simulink subsystem "BatteryHVElectrical_refsub"  (R2022a)
settings: Solver=VariableStepAuto  StartTime=0.0  StopTime=10.0  RelTol=1e-3
undefined symbols (not defined in the file): batteryHighVoltage, Minus, Plus
libraries: fl_lib x7, nesl_utility x6, ee_lib x1
settings Model: Creator=isaacito  LastModifiedBy=isaacito
settings SolverCC: AlgebraicLoopSolver=TrustRegion
settings DebuggingCC: UnconnectedInputMsg=warning  UnconnectedOutputMsg=warning  UnconnectedLineMsg=warning  SFMachineParentedDataDiag=warning
settings RTWCC: DLArmComputeVersion=19.05

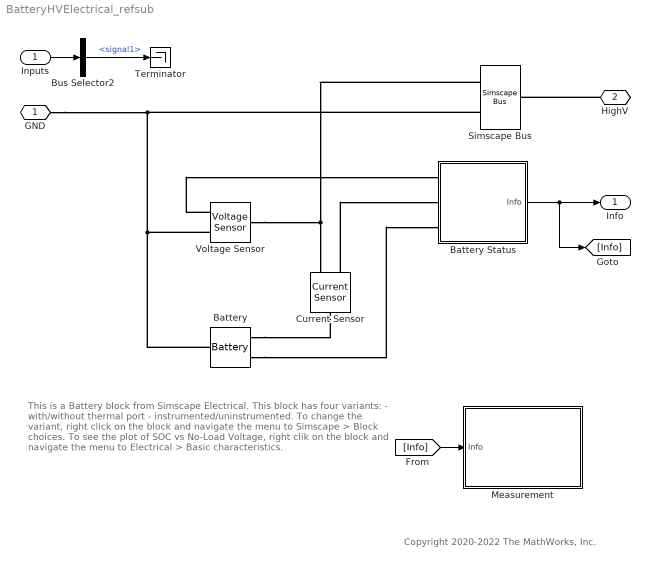
== system BatteryHVElectrical_refsub ==
  note: This is a Battery block from Simscape Electrical.
      | This block has four variants:
      | - with/without thermal port
      | - instrumented/uninstrumented.
      | To change the variant, right click on the block and
      | navigate the menu to Simscape > Block choices.
      |
      | To see the plot of SOC vs No-Load Voltage,
      | right clik on the block and navigate the menu
      | to Electrical > Basic characteristics.
  note: Copyright 2020-2022 The MathWorks, Inc.
  Inputs : Inport
  Battery : ee_lib/Sources/Battery  Vnom=batteryHighVoltage.packVoltage_V V  prm_dir=1  R1_dis=2 Ohm  R1_ch=2 Ohm  R1=batteryHighVoltage.internalResistance_Ohm Ohm  prm_AH=2  AH=batteryHighVoltage.nominalCharge_Ah hr*A  V1=batteryHighVoltage.packVoltage_V * 0.9 V  AH1=batteryHighVoltage.nominalCharge_Ah *0.5 hr*A  prm_R2=1  R2=2000 Ohm  prm_dyn=1  Rp1=0.005 Ohm  tau1=30 s  Rp2=0.005 Ohm  tau2=30 s  Rp3=0.005 Ohm  tau3=30 s  Rp4=0.005 Ohm  tau4=30 s  Rp5=0.005 Ohm  tau5=30 s  prm_fade=1  N_fade=100  AH_fade=45 hr*A  R1_fade=2.02 Ohm  R1_ch_fade=2.02 Ohm  V1_fade=10.35 V  prm_age=1  prm_age_OCV=1  OCV_age=0.9  SOC_age=60  delta_time_age_vec=[0] d  temperature_age_vec=[273] K  OCV_scaling_age=2.2134e6  OCV_offset_age=1.632e6  temp_exp_age=0.515833569 V  t_exp_age=0.75  i_specify=off  i_priority=None  i=0 A  i_nominal_specify=off  i_nominal_unit=A  i_nominal_value=1  v_specify=off  v_priority=None  v=0 V  v_nominal_specify=off  v_nominal_unit=V  v_nominal_value=1  charge_specify=on  charge_priority=High  charge=initial.hvBatteryCharge_Ah hr*A  charge_nominal_specify=off  charge_nominal_unit=hr*A  charge_nominal_value=1  num_cycles_specify=off  num_cycles_priority=High  num_cycles=0  num_cycles_nominal_specify=off  num_cycles_nominal_unit=1  num_cycles_nominal_value=1  Tmeas=298.15 K  Tmeas_age=298.15 K  Vnom_T2=batteryHighVoltage.packVoltage_V * 0.96 V  R1_T2=2 Ohm  R1_T2_dis=2.2 Ohm  R1_T2_ch=2.2 Ohm  V1_T2=batteryHighVoltage.packVoltage_V * 0.8 V  R2_T2=2200 Ohm  Rp1_T2=0.005 Ohm  tau1_T2=30 s  Rp2_T2=0.005 Ohm  tau2_T2=30 s  Rp3_T2=0.005 Ohm  tau3_T2=30 s  Rp4_T2=0.005 Ohm  tau4_T2=30 s  Rp5_T2=0.005 Ohm  tau5_T2=30 s  Tmeas2=273.15 K  thermal_mass=30 kJ/K  temperature_specify=off  temperature_priority=High  temperature=298.15 K  temperature_nominal_specify=off  temperature_nominal_unit=K  temperature_nominal_value=1
      settings: InternalSimscapePortConfiguration="{\"Bottom\":[],\"Left\":[{\"id\":\"p\",\"label\":\"+\",\"type\":\"foundation.electrical.electrical\"},{\"id\":\"q\",\"label\":\"q\",\"type\":\"output\"}],\"Right\":[{\"id\":\"n\",\"label\":\"-\",\"type\":\"foundation.electrical.electrical\"}],\"Top\":[]}"
  Battery Status : Subsystem
  Bus Selector2 : BusSelector  OutputSignals=signal1
  Current Sensor : fl_lib/Electrical/Electrical Sensors/Current Sensor
      settings: SourceProductBaseCode=PW,SS,VE
  Measurement : Subsystem
  Simscape Bus : SimscapeBus  HierarchyStrings=Plus;Minus
  Terminator : Terminator
  Voltage Sensor : fl_lib/Electrical/Electrical Sensors/Voltage Sensor
      settings: SourceProductBaseCode=PW,SS,VE
  GND : PMIOPort  Side=Left
  HighV : PMIOPort  Port=2  Side=Right
  Info : Outport
  wires:
  Battery Status/1(Info) -> Info/1, [Info]
  [Info] -> Measurement/1(Info)
  Bus Selector2/1 -> Terminator/1  "<signal1>"
  Inputs/1 -> Bus Selector2/1
  connections:
  Voltage Sensor/RConn2 -- GND/RConn1 -- Simscape Bus/LConn2 -- Battery/RConn1
  Voltage Sensor/LConn1 -- Simscape Bus/LConn1 -- Current Sensor/RConn2
  Current Sensor/RConn1 -- Battery Status/LConn2
  Voltage Sensor/RConn1 -- Battery Status/LConn1
  HighV/RConn1 -- Simscape Bus/RConn1
  Battery/LConn1 -- Current Sensor/LConn1
  Battery/LConn2 -- Battery Status/LConn3

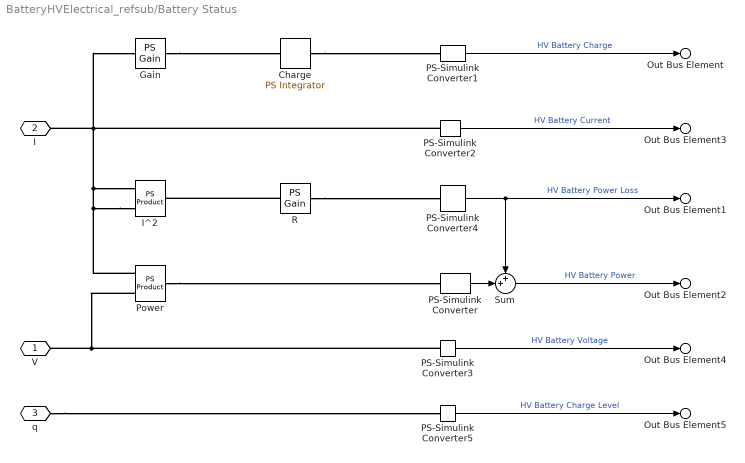
== system BatteryHVElectrical_refsub/Battery Status ==
  Charge : fl_lib/Physical Signals/Linear Operators/PS Integrator  reset_method=foundation.enum.IntegratorResetSpec.None  initial_condition_spec=foundation.enum.IntegratorICSpec.Internal  x0=initial.hvBatteryCharge_Ah A*hr
      settings: AttributesFormatString=%<x0> [%<x0_unit>]  SourceProductBaseCode=PW,SS,VE
  Gain : fl_lib/Physical Signals/Functions/PS Gain  gain=-1
      settings: AttributesFormatString=%<gain>  SourceProductBaseCode=PW,SS,VE
  I^2 : fl_lib/Physical Signals/Functions/PS Product
      settings: SourceProductBaseCode=PW,SS,VE
  PS-Simulink Converter : nesl_utility/PS-Simulink Converter  PhysicalDomain=network_engine_domain  SubClassName=ps_output  LeftPortType=input  RightPortType=output  PseudoPeriodic=off  Frequencies=[]  VectorFormat=1-D array  Unit=kW  AffineConversion=off
      settings: SourceProductBaseCode=SS,PW,VE
  PS-Simulink Converter1 : nesl_utility/PS-Simulink Converter  PhysicalDomain=network_engine_domain  SubClassName=ps_output  LeftPortType=input  RightPortType=output  PseudoPeriodic=off  Frequencies=[]  VectorFormat=1-D array  Unit=A*hr  AffineConversion=off
      settings: SourceProductBaseCode=SS,PW,VE
  PS-Simulink Converter2 : nesl_utility/PS-Simulink Converter  PhysicalDomain=network_engine_domain  SubClassName=ps_output  LeftPortType=input  RightPortType=output  PseudoPeriodic=off  Frequencies=[]  VectorFormat=1-D array  Unit=A  AffineConversion=off
      settings: SourceProductBaseCode=SS,PW,VE
  PS-Simulink Converter3 : nesl_utility/PS-Simulink Converter  PhysicalDomain=network_engine_domain  SubClassName=ps_output  LeftPortType=input  RightPortType=output  PseudoPeriodic=off  Frequencies=[]  VectorFormat=1-D array  Unit=V  AffineConversion=off
      settings: SourceProductBaseCode=SS,PW,VE
  PS-Simulink Converter4 : nesl_utility/PS-Simulink Converter  PhysicalDomain=network_engine_domain  SubClassName=ps_output  LeftPortType=input  RightPortType=output  PseudoPeriodic=off  Frequencies=[]  VectorFormat=1-D array  Unit=kW  AffineConversion=off
      settings: SourceProductBaseCode=SS,PW,VE
  PS-Simulink Converter5 : nesl_utility/PS-Simulink Converter  PhysicalDomain=network_engine_domain  SubClassName=ps_output  LeftPortType=input  RightPortType=output  PseudoPeriodic=off  Frequencies=[]  VectorFormat=1-D array  Unit=1  AffineConversion=off
      settings: SourceProductBaseCode=SS,PW,VE
  Power : fl_lib/Physical Signals/Functions/PS Product
      settings: SourceProductBaseCode=PW,SS,VE
  R : fl_lib/Physical Signals/Functions/PS Gain  gain=batteryHighVoltage.internal_R_Ohm Ohm
      settings: AttributesFormatString=%<gain> [%<gain_unit>]  SourceProductBaseCode=PW,SS,VE
  Sum : Sum  Inputs=++|
  V : PMIOPort  Side=Left
  I : PMIOPort  Port=2  Side=Left
  q : PMIOPort  Port=3  Side=Left
  Out Bus Element : Outport  PortName=Info  Element=Charge
      settings: AttributesFormatString=%<Unit>
  Out Bus Element3 : Outport  PortName=Info  Element=Current
      settings: AttributesFormatString=%<Unit>
  Out Bus Element1 : Outport  PortName=Info  Element=PowerLoss
      settings: AttributesFormatString=%<Unit>
  Out Bus Element2 : Outport  PortName=Info  Element=Power
      settings: AttributesFormatString=%<Unit>
  Out Bus Element4 : Outport  PortName=Info  Element=Voltage
      settings: AttributesFormatString=%<Unit>
  Out Bus Element5 : Outport  PortName=Info  Element=q
      settings: AttributesFormatString=%<Unit>
  wires:
  PS-Simulink Converter5/1 -> Out Bus Element5/1  "HV Battery Charge Level"
  PS-Simulink Converter3/1 -> Out Bus Element4/1  "HV Battery Voltage"
  PS-Simulink Converter2/1 -> Out Bus Element3/1  "HV Battery Current"
  PS-Simulink Converter/1 -> Sum/2
  Sum/1 -> Out Bus Element2/1  "HV Battery Power"
  PS-Simulink Converter1/1 -> Out Bus Element/1  "HV Battery Charge"
  PS-Simulink Converter4/1 -> Sum/1, Out Bus Element1/1  "HV Battery Power Loss"
  connections:
  q/RConn1 -- PS-Simulink Converter5/LConn1
  Power/LConn1 -- PS-Simulink Converter3/LConn1 -- V/RConn1
  Gain/RConn1 -- Charge/LConn1
  Charge/RConn1 -- PS-Simulink Converter1/LConn1
  Power/RConn1 -- PS-Simulink Converter/LConn1
  I^2/LConn1 -- Power/LConn2 -- I^2/LConn2 -- Gain/LConn1 -- I/RConn1 -- PS-Simulink Converter2/LConn1
  R/LConn1 -- I^2/RConn1
  R/RConn1 -- PS-Simulink Converter4/LConn1

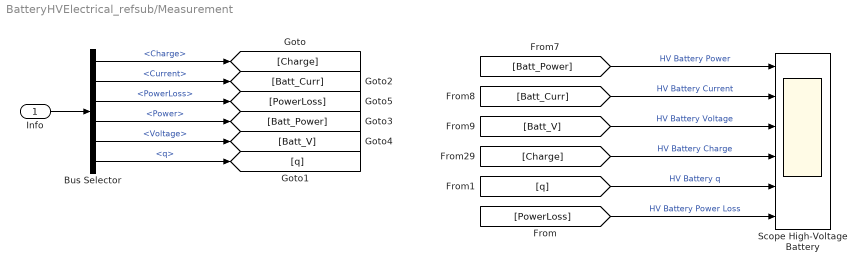
== system BatteryHVElectrical_refsub/Measurement ==
  Info : Inport
  Bus Selector : BusSelector  OutputSignals=Charge,Current,PowerLoss,Power,Voltage,q
  Scope High-Voltage Battery : Scope  NumInputPorts=6
  wires:
  [PowerLoss] -> Scope High-Voltage Battery/6  "HV Battery Power Loss"
  [q] -> Scope High-Voltage Battery/5  "HV Battery q"
  [Charge] -> Scope High-Voltage Battery/4  "HV Battery Charge"
  [Batt_V] -> Scope High-Voltage Battery/3  "HV Battery Voltage"
  [Batt_Curr] -> Scope High-Voltage Battery/2  "HV Battery Current"
  [Batt_Power] -> Scope High-Voltage Battery/1  "HV Battery Power"
  Bus Selector/6 -> [q]  "<q>"
  Bus Selector/5 -> [Batt_V]  "<Voltage>"
  Bus Selector/4 -> [Batt_Power]  "<Power>"
  Bus Selector/3 -> [PowerLoss]  "<PowerLoss>"
  Bus Selector/2 -> [Batt_Curr]  "<Current>"
  Bus Selector/1 -> [Charge]  "<Charge>"
  Info/1 -> Bus Selector/1
